simulink model "ControlComparison"  (R2018a)
settings: Solver=VariableStepAuto  StartTime=0  StopTime=4  FixedStep=1e-6
undefined symbols (not defined in the file): alternator, electrical_load, i_f_max, iceToAltRotRatio, n_ice_f, n_ice_i, normalizationFactor, rectifier, t_brake_f, t_brake_i, T_k, T_s
libraries: elec_lib x36, fl_lib x29, nesl_utility x26, neural x25, simulink x6, SimscapeCustomBlocks_lib x2
(part 2 of 3)

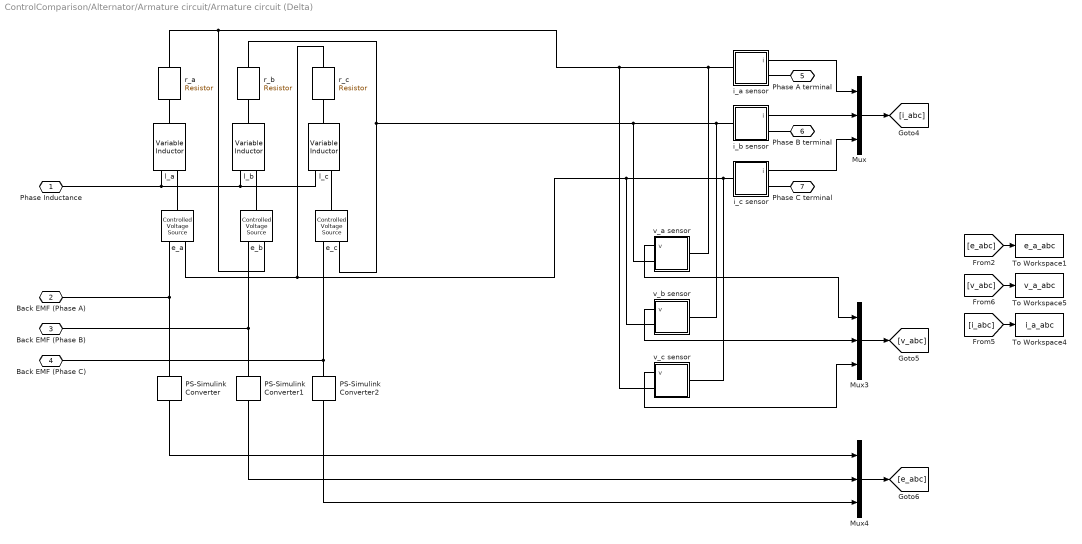
== system ControlComparison/Alternator/Armature circuit/Armature circuit (Delta) ==
  Mux : Mux  Inputs=3
  Mux3 : Mux  Inputs=3
  Mux4 : Mux  Inputs=3
  PS-Simulink Converter : nesl_utility/PS-Simulink Converter  PhysicalDomain=network_engine_domain  SubClassName=ps_output  LeftPortType=input  RightPortType=output  PseudoPeriodic=off  Frequencies=[]  Unit=1  AffineConversion=off
  PS-Simulink Converter1 : nesl_utility/PS-Simulink Converter  PhysicalDomain=network_engine_domain  SubClassName=ps_output  LeftPortType=input  RightPortType=output  PseudoPeriodic=off  Frequencies=[]  Unit=1  AffineConversion=off
  PS-Simulink Converter2 : nesl_utility/PS-Simulink Converter  PhysicalDomain=network_engine_domain  SubClassName=ps_output  LeftPortType=input  RightPortType=output  PseudoPeriodic=off  Frequencies=[]  Unit=1  AffineConversion=off
  To Workspace1 : ToWorkspace  VariableName=e_a_abc  SaveFormat=Timeseries  SampleTime=-1
  To Workspace4 : ToWorkspace  VariableName=i_a_abc  SaveFormat=Timeseries  SampleTime=-1
  To Workspace5 : ToWorkspace  VariableName=v_a_abc  SaveFormat=Timeseries  SampleTime=-1
  e_a : fl_lib/Electrical/Electrical Sources/Controlled Voltage Source
  e_b : fl_lib/Electrical/Electrical Sources/Controlled Voltage Source
  e_c : fl_lib/Electrical/Electrical Sources/Controlled Voltage Source
  i_a sensor : Subsystem
  i_b sensor : Subsystem
  i_c sensor : Subsystem
  l_a : elec_lib/Passive Devices/Variable Inductor  prm=1  Lmin=1e-6 H  g=1e-9 1/Ohm  i0=0 A  phi0=0 Wb
      settings: SourceProductName=Simscape Electronics  SourceProductBaseCode=SN
  l_b : elec_lib/Passive Devices/Variable Inductor  prm=1  Lmin=1e-6 H  g=1e-9 1/Ohm  i0=0 A  phi0=0 Wb
      settings: SourceProductName=Simscape Electronics  SourceProductBaseCode=SN
  l_c : elec_lib/Passive Devices/Variable Inductor  prm=1  Lmin=1e-6 H  g=1e-9 1/Ohm  i0=0 A  phi0=0 Wb
      settings: SourceProductName=Simscape Electronics  SourceProductBaseCode=SN
  r_a : elec_lib/Passive Devices/Resistor  R=alternator.stator.r.value Ohm  R_tol=5  enable_R_tol=0  tol_distribution=1  nSigma=4  enable_operating_limits=0  operating_limit_action=2  max_working_voltage=100 V  power_rating=1 W  enable_faults=0  fault_action=1  R_faulted=inf Ohm  enable_temporal_fault=0  t_fault=1 s  enable_behavioral_fault=0  max_permissible_current=1 A  t_fail_on_current=1 s  noise_mode=0  sample_time=1e-3 s  repeatability=1  auto_seed=4144164703  user_seed=0  Tdevice=25 degC  alpha=3.93e-3 1/K  Tmeas=25 degC  thermal_mass=100 J/K  power_derating_T1=70 degC  power_derating_T2=155 degC  operating_temperature_range_vec=[-50, 150] degC  temperature_specify=off  temperature_priority=High  temperature=298.15 K  temperature_nominal_specify=off  temperature_nominal_unit=K  temperature_nominal_value=1
  r_b : elec_lib/Passive Devices/Resistor  R=alternator.stator.r.value Ohm  R_tol=5  enable_R_tol=0  tol_distribution=1  nSigma=4  enable_operating_limits=0  operating_limit_action=2  max_working_voltage=100 V  power_rating=1 W  enable_faults=0  fault_action=1  R_faulted=inf Ohm  enable_temporal_fault=0  t_fault=1 s  enable_behavioral_fault=0  max_permissible_current=1 A  t_fail_on_current=1 s  noise_mode=0  sample_time=1e-3 s  repeatability=1  auto_seed=676943032  user_seed=0  Tdevice=25 degC  alpha=3.93e-3 1/K  Tmeas=25 degC  thermal_mass=100 J/K  power_derating_T1=70 degC  power_derating_T2=155 degC  operating_temperature_range_vec=[-50, 150] degC  temperature_specify=off  temperature_priority=High  temperature=298.15 K  temperature_nominal_specify=off  temperature_nominal_unit=K  temperature_nominal_value=1
  r_c : elec_lib/Passive Devices/Resistor  R=alternator.stator.r.value Ohm  R_tol=5  enable_R_tol=0  tol_distribution=1  nSigma=4  enable_operating_limits=0  operating_limit_action=2  max_working_voltage=100 V  power_rating=1 W  enable_faults=0  fault_action=1  R_faulted=inf Ohm  enable_temporal_fault=0  t_fault=1 s  enable_behavioral_fault=0  max_permissible_current=1 A  t_fail_on_current=1 s  noise_mode=0  sample_time=1e-3 s  repeatability=1  auto_seed=4168664255  user_seed=0  Tdevice=25 degC  alpha=3.93e-3 1/K  Tmeas=25 degC  thermal_mass=100 J/K  power_derating_T1=70 degC  power_derating_T2=155 degC  operating_temperature_range_vec=[-50, 150] degC  temperature_specify=off  temperature_priority=High  temperature=298.15 K  temperature_nominal_specify=off  temperature_nominal_unit=K  temperature_nominal_value=1
  v_a sensor : Subsystem
  v_b sensor : Subsystem
  v_c sensor : Subsystem
  Phase Inductance : PMIOPort  Side=Left
  Back EMF (Phase A) : PMIOPort  Port=2  Side=Left
  Back EMF (Phase B) : PMIOPort  Port=3  Side=Left
  Back EMF (Phase C) : PMIOPort  Port=4  Side=Left
  Phase A terminal : PMIOPort  Port=5  Side=Right
  Phase B terminal : PMIOPort  Port=6  Side=Right
  Phase C terminal : PMIOPort  Port=7  Side=Right
  wires:
  i_a sensor/1(i) -> Mux/1
  i_b sensor/1(i) -> Mux/2
  i_c sensor/1(i) -> Mux/3
  Mux/1 -> [i_abc]
  Mux3/1 -> [v_abc]
  v_b sensor/1(v) -> Mux3/2
  v_c sensor/1(v) -> Mux3/3
  v_a sensor/1(v) -> Mux3/1
  [i_abc] -> To Workspace4/1
  [v_abc] -> To Workspace5/1
  PS-Simulink Converter/1 -> Mux4/1
  PS-Simulink Converter1/1 -> Mux4/2
  PS-Simulink Converter2/1 -> Mux4/3
  Mux4/1 -> [e_abc]
  [e_abc] -> To Workspace1/1
  connections:
  i_a sensor/RConn1 -- Phase A terminal/RConn1
  Back EMF (Phase A)/RConn1 -- e_a/RConn1 -- PS-Simulink Converter/LConn1
  Back EMF (Phase B)/RConn1 -- e_b/RConn1 -- PS-Simulink Converter1/LConn1
  Back EMF (Phase C)/RConn1 -- e_c/RConn1 -- PS-Simulink Converter2/LConn1
  e_c/LConn1 -- l_c/LConn2
  e_b/LConn1 -- l_b/LConn2
  e_a/LConn1 -- l_a/LConn2
  r_c/LConn1 -- l_c/RConn1
  r_b/LConn1 -- l_b/RConn1
  r_a/LConn1 -- l_a/RConn1
  i_c sensor/RConn1 -- Phase C terminal/RConn1
  i_b sensor/RConn1 -- Phase B terminal/RConn1
  l_a/LConn1 -- Phase Inductance/RConn1 -- l_b/LConn1 -- l_c/LConn1
  e_b/RConn2 -- r_a/RConn1 -- v_a sensor/LConn1 -- i_a sensor/LConn1 -- v_c sensor/RConn1
  v_a sensor/RConn1 -- e_c/RConn2 -- r_b/RConn1 -- i_b sensor/LConn1 -- v_b sensor/LConn1
  r_c/RConn1 -- e_a/RConn2 -- v_c sensor/LConn1 -- i_c sensor/LConn1 -- v_b sensor/RConn1

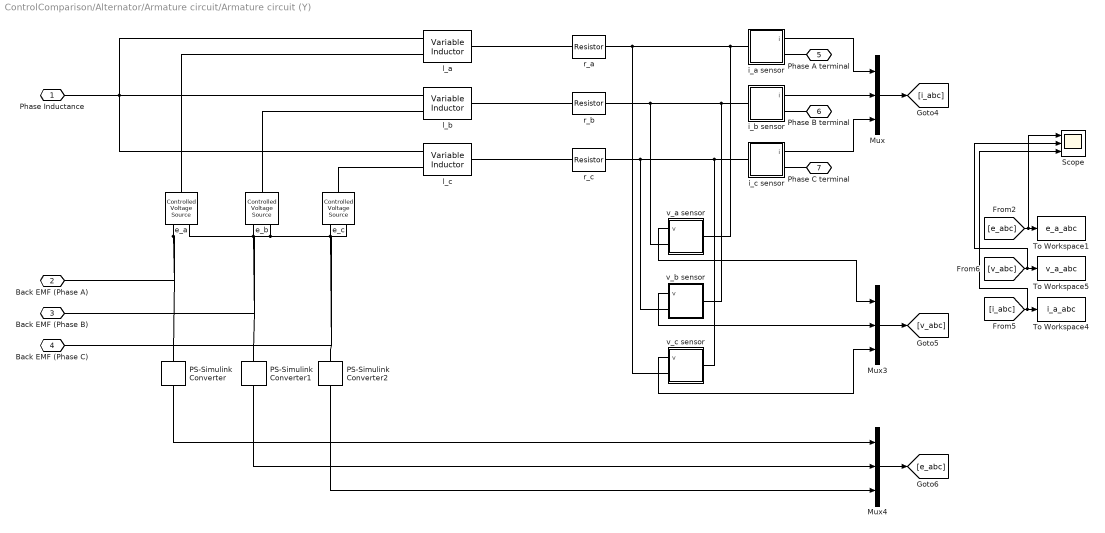
== system ControlComparison/Alternator/Armature circuit/Armature circuit (Y) ==
  Mux : Mux  Inputs=3
  Mux3 : Mux  Inputs=3
  Mux4 : Mux  Inputs=3
  PS-Simulink Converter : nesl_utility/PS-Simulink Converter  PhysicalDomain=network_engine_domain  SubClassName=ps_output  LeftPortType=input  RightPortType=output  PseudoPeriodic=off  Frequencies=[]  Unit=1  AffineConversion=off
  PS-Simulink Converter1 : nesl_utility/PS-Simulink Converter  PhysicalDomain=network_engine_domain  SubClassName=ps_output  LeftPortType=input  RightPortType=output  PseudoPeriodic=off  Frequencies=[]  Unit=1  AffineConversion=off
  PS-Simulink Converter2 : nesl_utility/PS-Simulink Converter  PhysicalDomain=network_engine_domain  SubClassName=ps_output  LeftPortType=input  RightPortType=output  PseudoPeriodic=off  Frequencies=[]  Unit=1  AffineConversion=off
  Scope : Scope  NumInputPorts=3
  To Workspace1 : ToWorkspace  VariableName=e_a_abc  SaveFormat=Timeseries  SampleTime=-1
  To Workspace4 : ToWorkspace  VariableName=i_a_abc  SaveFormat=Timeseries  SampleTime=-1
  To Workspace5 : ToWorkspace  VariableName=v_a_abc  SaveFormat=Timeseries  SampleTime=-1
  e_a : fl_lib/Electrical/Electrical Sources/Controlled Voltage Source
  e_b : fl_lib/Electrical/Electrical Sources/Controlled Voltage Source
  e_c : fl_lib/Electrical/Electrical Sources/Controlled Voltage Source
  i_a sensor : Subsystem
  i_b sensor : Subsystem
  i_c sensor : Subsystem
  l_a : elec_lib/Passive Devices/Variable Inductor  prm=1  Lmin=1e-6 H  g=1e-9 1/Ohm  i0=0 A  phi0=0 Wb
      settings: SourceProductName=Simscape Electronics  SourceProductBaseCode=SN
  l_b : elec_lib/Passive Devices/Variable Inductor  prm=1  Lmin=1e-6 H  g=1e-9 1/Ohm  i0=0 A  phi0=0 Wb
      settings: SourceProductName=Simscape Electronics  SourceProductBaseCode=SN
  l_c : elec_lib/Passive Devices/Variable Inductor  prm=1  Lmin=1e-6 H  g=1e-9 1/Ohm  i0=0 A  phi0=0 Wb
      settings: SourceProductName=Simscape Electronics  SourceProductBaseCode=SN
  r_a : elec_lib/Passive Devices/Resistor  R=alternator.stator.r.value/3 Ohm  R_tol=5  enable_R_tol=0  tol_distribution=1  nSigma=4  enable_operating_limits=0  operating_limit_action=2  max_working_voltage=100 V  power_rating=1 W  enable_faults=0  fault_action=1  R_faulted=inf Ohm  enable_temporal_fault=0  t_fault=1 s  enable_behavioral_fault=0  max_permissible_current=1 A  t_fail_on_current=1 s  noise_mode=0  sample_time=1e-3 s  repeatability=1  auto_seed=3922919431  user_seed=0  Tdevice=25 degC  alpha=3.93e-3 1/K  Tmeas=25 degC  thermal_mass=100 J/K  power_derating_T1=70 degC  power_derating_T2=155 degC  operating_temperature_range_vec=[-50, 150] degC  temperature_specify=off  temperature_priority=High  temperature=298.15 K  temperature_nominal_specify=off  temperature_nominal_unit=K  temperature_nominal_value=1
  r_b : elec_lib/Passive Devices/Resistor  R=alternator.stator.r.value/3 Ohm  R_tol=5  enable_R_tol=0  tol_distribution=1  nSigma=4  enable_operating_limits=0  operating_limit_action=2  max_working_voltage=100 V  power_rating=1 W  enable_faults=0  fault_action=1  R_faulted=inf Ohm  enable_temporal_fault=0  t_fault=1 s  enable_behavioral_fault=0  max_permissible_current=1 A  t_fail_on_current=1 s  noise_mode=0  sample_time=1e-3 s  repeatability=1  auto_seed=2715962282  user_seed=0  Tdevice=25 degC  alpha=3.93e-3 1/K  Tmeas=25 degC  thermal_mass=100 J/K  power_derating_T1=70 degC  power_derating_T2=155 degC  operating_temperature_range_vec=[-50, 150] degC  temperature_specify=off  temperature_priority=High  temperature=298.15 K  temperature_nominal_specify=off  temperature_nominal_unit=K  temperature_nominal_value=1
  r_c : elec_lib/Passive Devices/Resistor  R=alternator.stator.r.value/3 Ohm  R_tol=5  enable_R_tol=0  tol_distribution=1  nSigma=4  enable_operating_limits=0  operating_limit_action=2  max_working_voltage=100 V  power_rating=1 W  enable_faults=0  fault_action=1  R_faulted=inf Ohm  enable_temporal_fault=0  t_fault=1 s  enable_behavioral_fault=0  max_permissible_current=1 A  t_fail_on_current=1 s  noise_mode=0  sample_time=1e-3 s  repeatability=1  auto_seed=418932850  user_seed=0  Tdevice=25 degC  alpha=3.93e-3 1/K  Tmeas=25 degC  thermal_mass=100 J/K  power_derating_T1=70 degC  power_derating_T2=155 degC  operating_temperature_range_vec=[-50, 150] degC  temperature_specify=off  temperature_priority=High  temperature=298.15 K  temperature_nominal_specify=off  temperature_nominal_unit=K  temperature_nominal_value=1
  v_a sensor : Subsystem
  v_b sensor : Subsystem
  v_c sensor : Subsystem
  Phase Inductance : PMIOPort  Side=Left
  Back EMF (Phase A) : PMIOPort  Port=2  Side=Left
  Back EMF (Phase B) : PMIOPort  Port=3  Side=Left
  Back EMF (Phase C) : PMIOPort  Port=4  Side=Left
  Phase A terminal : PMIOPort  Port=5  Side=Right
  Phase B terminal : PMIOPort  Port=6  Side=Right
  Phase C terminal : PMIOPort  Port=7  Side=Right
  wires:
  i_a sensor/1(i) -> Mux/1
  i_b sensor/1(i) -> Mux/2
  i_c sensor/1(i) -> Mux/3
  Mux/1 -> [i_abc]
  Mux3/1 -> [v_abc]
  v_b sensor/1(v) -> Mux3/2
  v_c sensor/1(v) -> Mux3/3
  v_a sensor/1(v) -> Mux3/1
  [i_abc] -> Scope/3, To Workspace4/1
  [v_abc] -> Scope/2, To Workspace5/1
  PS-Simulink Converter/1 -> Mux4/1
  PS-Simulink Converter1/1 -> Mux4/2
  PS-Simulink Converter2/1 -> Mux4/3
  Mux4/1 -> [e_abc]
  [e_abc] -> Scope/1, To Workspace1/1
  connections:
  i_a sensor/RConn1 -- Phase A terminal/RConn1
  e_a/RConn2 -- e_c/RConn2 -- e_b/RConn2
  e_c/LConn1 -- l_c/LConn2
  e_b/LConn1 -- l_b/LConn2
  e_a/LConn1 -- l_a/LConn2
  r_c/LConn1 -- l_c/RConn1
  r_b/LConn1 -- l_b/RConn1
  r_a/LConn1 -- l_a/RConn1
  i_a sensor/LConn1 -- v_a sensor/LConn1 -- v_c sensor/RConn1 -- r_a/RConn1
  i_c sensor/RConn1 -- Phase C terminal/RConn1
  i_b sensor/RConn1 -- Phase B terminal/RConn1
  i_c sensor/LConn1 -- v_c sensor/LConn1 -- v_b sensor/RConn1 -- r_c/RConn1
  r_b/RConn1 -- v_a sensor/RConn1 -- v_b sensor/LConn1 -- i_b sensor/LConn1
  l_a/LConn1 -- Phase Inductance/RConn1 -- l_c/LConn1 -- l_b/LConn1
  e_a/RConn1 -- Back EMF (Phase A)/RConn1 -- PS-Simulink Converter/LConn1
  e_b/RConn1 -- Back EMF (Phase B)/RConn1 -- PS-Simulink Converter1/LConn1
  e_c/RConn1 -- Back EMF (Phase C)/RConn1 -- PS-Simulink Converter2/LConn1

== system ControlComparison/Alternator/Excitation circuit/Current sensor ==
  Current Sensor1 : fl_lib/Electrical/Electrical Sensors/Current Sensor
  PS-Simulink Converter1 : nesl_utility/PS-Simulink Converter  PhysicalDomain=network_engine_domain  SubClassName=ps_output  LeftPortType=input  RightPortType=output  PseudoPeriodic=off  Frequencies=[]  Unit=1  AffineConversion=off
  Sample delay : TransferFcn  Denominator=[T_s 1]
  + : PMIOPort  Side=Left
  - : PMIOPort  Port=2  Side=Right
  i (PS) : PMIOPort  Port=3  Side=Right
  i (Sim) : Outport
  wires:
  Sample delay/1 -> i (Sim)/1
  PS-Simulink Converter1/1 -> Sample delay/1
  connections:
  Current Sensor1/RConn2 -- -/RConn1
  Current Sensor1/LConn1 -- +/RConn1
  PS-Simulink Converter1/LConn1 -- i (PS)/RConn1 -- Current Sensor1/RConn1

== system ControlComparison/Alternator/Excitation circuit/Driver ==
  Controlled PWM Voltage : elec_lib/Actuators & Drivers/Drivers/Controlled PWM Voltage  F=alternator.rotor.control.pwm.f_s Hz  TD=0 s  pulse_width_offset=0 s  pulse_min=0 s  Vmin=0 V  Vmax=5 V  Vm=5 V  pwm_or_av=1  event_type=2  sample_time=T_s s  u_min=0  u_max=1
      settings: SourceProductName=Simscape Electronics  SourceProductBaseCode=SN  LogSimulationData=on
  Electrical Reference : fl_lib/Electrical/Electrical Elements/Electrical Reference
  Gate Driver : elec_lib/Actuators & Drivers/Drivers/Gate Driver  vHigh=rectifier.s.v_gs_on*1.5 V  vLow=0 V  parameterization=1  rHigh=100 Ohm  rLow=10 Ohm  tRise=20 ns  tFall=20 ns  cLoad=10 nF  enable_faults=0  t_fault=1 s  fault_type=1  uHighValue=0.7  uLowValue=0.3  tHigh=50 ns  tLow=100 ns  ZonTime_specify=off  ZonTime_priority=None  ZonTime=0 s  ZoffTime_specify=off  ZoffTime_priority=None  ZoffTime=0 s  uHigh=2.0 V  uLow=0.8 V
      settings: SourceProductName=Simscape Electronics  SourceProductBaseCode=SN  LogSimulationData=on
  d : PMIOPort  Side=Left
  v_g : PMIOPort  Port=2  Side=Right
  v_s : PMIOPort  Port=3  Side=Right
  connections:
  Gate Driver/LConn2 -- Electrical Reference/LConn1 -- Controlled PWM Voltage/RConn2
  Controlled PWM Voltage/RConn1 -- Gate Driver/LConn1
  v_g/RConn1 -- Gate Driver/RConn1
  v_s/RConn1 -- Gate Driver/RConn2
  d/RConn1 -- Controlled PWM Voltage/LConn1

== system ControlComparison/Control scheme/Conventional Control Scheme/Excitation current controller ==
  e : Inport
  on : Inport  Port=2
  Constant : Constant
  Fcn : Fcn  Expr=u > 0
  Switch : Switch  Criteria=u2 > Threshold  Threshold=0.5
  u : Outport
  wires:
  Switch/1 -> u/1
  on/1 -> Switch/2
  Constant/1 -> Switch/3
  Fcn/1 -> Switch/1
  e/1 -> Fcn/1

== system ControlComparison/Control scheme/Full Excitation Current Control Scheme/Excitation current controller ==
  e : Inport
  on : Inport  Port=2
  Constant : Constant
  Fcn : Fcn  Expr=u > 0
  Switch : Switch  Criteria=u2 > Threshold  Threshold=0.5
  u : Outport
  wires:
  Switch/1 -> u/1
  on/1 -> Switch/2
  Constant/1 -> Switch/3
  Fcn/1 -> Switch/1
  e/1 -> Fcn/1

== system ControlComparison/Control scheme/Neural MPPT Control Scheme/Excitation current controller ==
  e : Inport
  on : Inport  Port=2
  Constant : Constant
  Fcn : Fcn  Expr=u > 0
  Switch : Switch  Criteria=u2 > Threshold  Threshold=0.5
  u : Outport
  wires:
  Switch/1 -> u/1
  on/1 -> Switch/2
  Constant/1 -> Switch/3
  Fcn/1 -> Switch/1
  e/1 -> Fcn/1

== system ControlComparison/Control scheme/Neural MPPT Control Scheme/Mapped Duty Cycle Neural Controller ==
  Input : Inport  PortDimensions=3
      mask Display: e = 0.06;c1 = [120 230 180]/255;c2 = ([120 230 180]+0)/(256+128);c3 = ([120 230 180]+128)/(256+128);patch([0 1 1 0],[0 0 1 1],c1);patch([0 1 1 1-e 1-e 0+e],[0 0 1 1-e 0+e 0+e],c2);patch([0 0 1 1-e 0+e 0+e],[0 1 1 1-e 1-e 0+e],c3);plot([0 1 1 0 0],[0 0 1 1 0]);
  Layer 1 : Subsystem
      mask Display: e = 0.06;c1 = [120 150 230]/255;c2 = ([120 150 230]+0)/383;c3 = ([120 150 230]+128)/383;patch([0 1 1 0],[0 0 1 1],c1);patch([0 1 1 1-e 1-e 0+e],[0 0 1 1-e 0+e 0+e],c2);patch([0 0 1 1-e 0+e 0+e],[0 1 1 1-e 1-e 0+e],c3);plot([0 1 1 0 0],[0 0 1 1 0]);
  Layer 2 : Subsystem
      mask Display: e = 0.06;c1 = [120 150 230]/255;c2 = ([120 150 230]+0)/383;c3 = ([120 150 230]+128)/383;patch([0 1 1 0],[0 0 1 1],c1);patch([0 1 1 1-e 1-e 0+e],[0 0 1 1-e 0+e 0+e],c2);patch([0 0 1 1-e 0+e 0+e],[0 1 1 1-e 1-e 0+e],c3);plot([0 1 1 0 0],[0 0 1 1 0]);
  Process Input 1 : Subsystem
      mask Display: e = 0.06;c1 = [120 150 230]/255;c2 = ([120 150 230]+0)/383;c3 = ([120 150 230]+128)/383;patch([0 1 1 0],[0 0 1 1],c1);patch([0 1 1 1-e 1-e 0+e],[0 0 1 1-e 0+e 0+e],c2);patch([0 0 1 1-e 0+e 0+e],[0 1 1 1-e 1-e 0+e],c3);plot([0 1 1 0 0],[0 0 1 1 0]);
  Process Output 1 : Subsystem
      mask Display: e = 0.06;c1 = [120 150 230]/255;c2 = ([120 150 230]+0)/383;c3 = ([120 150 230]+128)/383;patch([0 1 1 0],[0 0 1 1],c1);patch([0 1 1 1-e 1-e 0+e],[0 0 1 1-e 0+e 0+e],c2);patch([0 0 1 1-e 0+e 0+e],[0 1 1 1-e 1-e 0+e],c3);plot([0 1 1 0 0],[0 0 1 1 0]);
  Output : Outport  InitialOutput=0
      mask Display: e = 0.06;c1 = [120 230 180]/255;c2 = ([120 230 180]+0)/(256+128);c3 = ([120 230 180]+128)/(256+128);patch([0 1 1 0],[0 0 1 1],c1);patch([0 1 1 1-e 1-e 0+e],[0 0 1 1-e 0+e 0+e],c2);patch([0 0 1 1-e 0+e 0+e],[0 1 1 1-e 1-e 0+e],c3);plot([0 1 1 0 0],[0 0 1 1 0]);
  wires:
  Layer 2/1("a{2}") -> Process Output 1/1(a)
  [feedback1] -> Layer 2/1("a{1} ")
  Layer 1/1("a{1}") -> [feedback1]
  Process Input 1/1(p) -> Layer 1/1("p{1}")
  Process Output 1/1(y) -> Output/1
  Input/1 -> Process Input 1/1(x)

== system ControlComparison/i_l sensor/Current Sensor/Ideal current sensor ==
  Current Sensor : fl_lib/Electrical/Electrical Sensors/Current Sensor
  PS-Simulink Converter : nesl_utility/PS-Simulink Converter  PhysicalDomain=network_engine_domain  SubClassName=ps_output  LeftPortType=input  RightPortType=output  PseudoPeriodic=off  Frequencies=[]  Unit=1  AffineConversion=off
  + : PMIOPort  Side=Left
  - : PMIOPort  Port=2  Side=Right
  i : Outport
  wires:
  PS-Simulink Converter/1 -> i/1
  connections:
  Current Sensor/RConn2 -- -/RConn1
  Current Sensor/LConn1 -- +/RConn1
  PS-Simulink Converter/LConn1 -- Current Sensor/RConn1

== system ControlComparison/i_l sensor/Current Sensor/Noise addition ==
  u : Inport
  Band-Limited White Noise : simulink/Sources/Band-Limited White Noise  Cov=[0.1]  Ts=T_s  seed=[seed]
  Gain : Gain  Gain=1/100
  Gain3 : Gain  Gain=noise
  Product2 : Product
  Sum1 : Sum  Inputs=|++
  Zero-Order Hold : ZeroOrderHold  SampleTime=T_s
  u + n : Outport
  wires:
  Gain3/1 -> Product2/1
  Product2/1 -> Sum1/1
  Gain/1 -> Product2/2
  u/1 -> Sum1/2, Gain3/1
  Band-Limited White Noise/1 -> Gain/1
  Sum1/1 -> Zero-Order Hold/1
  Zero-Order Hold/1 -> u + n/1

== system ControlComparison/v_b sensor/Voltage Sensor/Ideal voltage sensor ==
  PS-Simulink Converter : nesl_utility/PS-Simulink Converter  PhysicalDomain=network_engine_domain  SubClassName=ps_output  LeftPortType=input  RightPortType=output  PseudoPeriodic=off  Frequencies=[]  Unit=1  AffineConversion=off
  Voltage Sensor : fl_lib/Electrical/Electrical Sensors/Voltage Sensor
  + : PMIOPort  Side=Left
  - : PMIOPort  Port=2  Side=Right
  v : Outport
  wires:
  PS-Simulink Converter/1 -> v/1
  connections:
  Voltage Sensor/LConn1 -- +/RConn1
  -/RConn1 -- Voltage Sensor/RConn2
  Voltage Sensor/RConn1 -- PS-Simulink Converter/LConn1

== system ControlComparison/v_b sensor/Voltage Sensor/Noise addition ==
  u : Inport
  Band-Limited White Noise : simulink/Sources/Band-Limited White Noise  Cov=[0.1]  Ts=T_s  seed=[seed]
  Gain : Gain  Gain=1/100
  Gain3 : Gain  Gain=noise
  Product2 : Product
  Sum1 : Sum  Inputs=|++
  Zero-Order Hold : ZeroOrderHold  SampleTime=T_s
  u + n : Outport
  wires:
  Gain3/1 -> Product2/1
  Product2/1 -> Sum1/1
  Gain/1 -> Product2/2
  u/1 -> Sum1/2, Gain3/1
  Band-Limited White Noise/1 -> Gain/1
  Sum1/1 -> Zero-Order Hold/1
  Zero-Order Hold/1 -> u + n/1

== system ControlComparison/v_l sensor/Voltage Sensor/Ideal voltage sensor ==
  PS-Simulink Converter : nesl_utility/PS-Simulink Converter  PhysicalDomain=network_engine_domain  SubClassName=ps_output  LeftPortType=input  RightPortType=output  PseudoPeriodic=off  Frequencies=[]  Unit=1  AffineConversion=off
  Voltage Sensor : fl_lib/Electrical/Electrical Sensors/Voltage Sensor
  + : PMIOPort  Side=Left
  - : PMIOPort  Port=2  Side=Right
  v : Outport
  wires:
  PS-Simulink Converter/1 -> v/1
  connections:
  Voltage Sensor/LConn1 -- +/RConn1
  -/RConn1 -- Voltage Sensor/RConn2
  Voltage Sensor/RConn1 -- PS-Simulink Converter/LConn1

== system ControlComparison/v_l sensor/Voltage Sensor/Noise addition ==
  u : Inport
  Band-Limited White Noise : simulink/Sources/Band-Limited White Noise  Cov=[0.1]  Ts=T_s  seed=[seed]
  Gain : Gain  Gain=1/100
  Gain3 : Gain  Gain=noise
  Product2 : Product
  Sum1 : Sum  Inputs=|++
  Zero-Order Hold : ZeroOrderHold  SampleTime=T_s
  u + n : Outport
  wires:
  Gain3/1 -> Product2/1
  Product2/1 -> Sum1/1
  Gain/1 -> Product2/2
  u/1 -> Sum1/2, Gain3/1
  Band-Limited White Noise/1 -> Gain/1
  Sum1/1 -> Zero-Order Hold/1
  Zero-Order Hold/1 -> u + n/1

== system ControlComparison/Alternator/Armature circuit/Armature circuit (Delta)/i_a sensor ==
  Current Sensor : fl_lib/Electrical/Electrical Sensors/Current Sensor
  PS-Simulink Converter : nesl_utility/PS-Simulink Converter  PhysicalDomain=network_engine_domain  SubClassName=ps_output  LeftPortType=input  RightPortType=output  PseudoPeriodic=off  Frequencies=[]  Unit=1  AffineConversion=off
  + : PMIOPort  Side=Left
  - : PMIOPort  Port=2  Side=Right
  i : Outport
  wires:
  PS-Simulink Converter/1 -> i/1
  connections:
  Current Sensor/RConn2 -- -/RConn1
  Current Sensor/LConn1 -- +/RConn1
  PS-Simulink Converter/LConn1 -- Current Sensor/RConn1

== system ControlComparison/Alternator/Armature circuit/Armature circuit (Delta)/i_b sensor ==
  Current Sensor : fl_lib/Electrical/Electrical Sensors/Current Sensor
  PS-Simulink Converter : nesl_utility/PS-Simulink Converter  PhysicalDomain=network_engine_domain  SubClassName=ps_output  LeftPortType=input  RightPortType=output  PseudoPeriodic=off  Frequencies=[]  Unit=1  AffineConversion=off
  + : PMIOPort  Side=Left
  - : PMIOPort  Port=2  Side=Right
  i : Outport
  wires:
  PS-Simulink Converter/1 -> i/1
  connections:
  Current Sensor/RConn2 -- -/RConn1
  Current Sensor/LConn1 -- +/RConn1
  PS-Simulink Converter/LConn1 -- Current Sensor/RConn1

== system ControlComparison/Alternator/Armature circuit/Armature circuit (Delta)/i_c sensor ==
  Current Sensor : fl_lib/Electrical/Electrical Sensors/Current Sensor
  PS-Simulink Converter : nesl_utility/PS-Simulink Converter  PhysicalDomain=network_engine_domain  SubClassName=ps_output  LeftPortType=input  RightPortType=output  PseudoPeriodic=off  Frequencies=[]  Unit=1  AffineConversion=off
  + : PMIOPort  Side=Left
  - : PMIOPort  Port=2  Side=Right
  i : Outport
  wires:
  PS-Simulink Converter/1 -> i/1
  connections:
  Current Sensor/RConn2 -- -/RConn1
  Current Sensor/LConn1 -- +/RConn1
  PS-Simulink Converter/LConn1 -- Current Sensor/RConn1

== system ControlComparison/Alternator/Armature circuit/Armature circuit (Delta)/v_a sensor ==
  PS-Simulink Converter : nesl_utility/PS-Simulink Converter  PhysicalDomain=network_engine_domain  SubClassName=ps_output  LeftPortType=input  RightPortType=output  PseudoPeriodic=off  Frequencies=[]  Unit=1  AffineConversion=off
  Voltage Sensor : fl_lib/Electrical/Electrical Sensors/Voltage Sensor
  + : PMIOPort  Side=Left
  - : PMIOPort  Port=2  Side=Right
  v : Outport
  wires:
  PS-Simulink Converter/1 -> v/1
  connections:
  Voltage Sensor/LConn1 -- +/RConn1
  -/RConn1 -- Voltage Sensor/RConn2
  Voltage Sensor/RConn1 -- PS-Simulink Converter/LConn1

== system ControlComparison/Alternator/Armature circuit/Armature circuit (Delta)/v_b sensor ==
  PS-Simulink Converter : nesl_utility/PS-Simulink Converter  PhysicalDomain=network_engine_domain  SubClassName=ps_output  LeftPortType=input  RightPortType=output  PseudoPeriodic=off  Frequencies=[]  Unit=1  AffineConversion=off
  Voltage Sensor : fl_lib/Electrical/Electrical Sensors/Voltage Sensor
  + : PMIOPort  Side=Left
  - : PMIOPort  Port=2  Side=Right
  v : Outport
  wires:
  PS-Simulink Converter/1 -> v/1
  connections:
  Voltage Sensor/LConn1 -- +/RConn1
  -/RConn1 -- Voltage Sensor/RConn2
  Voltage Sensor/RConn1 -- PS-Simulink Converter/LConn1

== system ControlComparison/Alternator/Armature circuit/Armature circuit (Delta)/v_c sensor ==
  PS-Simulink Converter : nesl_utility/PS-Simulink Converter  PhysicalDomain=network_engine_domain  SubClassName=ps_output  LeftPortType=input  RightPortType=output  PseudoPeriodic=off  Frequencies=[]  Unit=1  AffineConversion=off
  Voltage Sensor : fl_lib/Electrical/Electrical Sensors/Voltage Sensor
  + : PMIOPort  Side=Left
  - : PMIOPort  Port=2  Side=Right
  v : Outport
  wires:
  PS-Simulink Converter/1 -> v/1
  connections:
  Voltage Sensor/LConn1 -- +/RConn1
  -/RConn1 -- Voltage Sensor/RConn2
  Voltage Sensor/RConn1 -- PS-Simulink Converter/LConn1

== system ControlComparison/Alternator/Armature circuit/Armature circuit (Y)/i_a sensor ==
  Current Sensor : fl_lib/Electrical/Electrical Sensors/Current Sensor
  PS-Simulink Converter : nesl_utility/PS-Simulink Converter  PhysicalDomain=network_engine_domain  SubClassName=ps_output  LeftPortType=input  RightPortType=output  PseudoPeriodic=off  Frequencies=[]  Unit=1  AffineConversion=off
  + : PMIOPort  Side=Left
  - : PMIOPort  Port=2  Side=Right
  i : Outport
  wires:
  PS-Simulink Converter/1 -> i/1
  connections:
  Current Sensor/RConn2 -- -/RConn1
  Current Sensor/LConn1 -- +/RConn1
  PS-Simulink Converter/LConn1 -- Current Sensor/RConn1

== system ControlComparison/Alternator/Armature circuit/Armature circuit (Y)/i_b sensor ==
  Current Sensor : fl_lib/Electrical/Electrical Sensors/Current Sensor
  PS-Simulink Converter : nesl_utility/PS-Simulink Converter  PhysicalDomain=network_engine_domain  SubClassName=ps_output  LeftPortType=input  RightPortType=output  PseudoPeriodic=off  Frequencies=[]  Unit=1  AffineConversion=off
  + : PMIOPort  Side=Left
  - : PMIOPort  Port=2  Side=Right
  i : Outport
  wires:
  PS-Simulink Converter/1 -> i/1
  connections:
  Current Sensor/RConn2 -- -/RConn1
  Current Sensor/LConn1 -- +/RConn1
  PS-Simulink Converter/LConn1 -- Current Sensor/RConn1

== system ControlComparison/Alternator/Armature circuit/Armature circuit (Y)/i_c sensor ==
  Current Sensor : fl_lib/Electrical/Electrical Sensors/Current Sensor
  PS-Simulink Converter : nesl_utility/PS-Simulink Converter  PhysicalDomain=network_engine_domain  SubClassName=ps_output  LeftPortType=input  RightPortType=output  PseudoPeriodic=off  Frequencies=[]  Unit=1  AffineConversion=off
  + : PMIOPort  Side=Left
  - : PMIOPort  Port=2  Side=Right
  i : Outport
  wires:
  PS-Simulink Converter/1 -> i/1
  connections:
  Current Sensor/RConn2 -- -/RConn1
  Current Sensor/LConn1 -- +/RConn1
  PS-Simulink Converter/LConn1 -- Current Sensor/RConn1

== system ControlComparison/Alternator/Armature circuit/Armature circuit (Y)/v_a sensor ==
  PS-Simulink Converter : nesl_utility/PS-Simulink Converter  PhysicalDomain=network_engine_domain  SubClassName=ps_output  LeftPortType=input  RightPortType=output  PseudoPeriodic=off  Frequencies=[]  Unit=1  AffineConversion=off
  Voltage Sensor : fl_lib/Electrical/Electrical Sensors/Voltage Sensor
  + : PMIOPort  Side=Left
  - : PMIOPort  Port=2  Side=Right
  v : Outport
  wires:
  PS-Simulink Converter/1 -> v/1
  connections:
  Voltage Sensor/LConn1 -- +/RConn1
  -/RConn1 -- Voltage Sensor/RConn2
  Voltage Sensor/RConn1 -- PS-Simulink Converter/LConn1

== system ControlComparison/Alternator/Armature circuit/Armature circuit (Y)/v_b sensor ==
  PS-Simulink Converter : nesl_utility/PS-Simulink Converter  PhysicalDomain=network_engine_domain  SubClassName=ps_output  LeftPortType=input  RightPortType=output  PseudoPeriodic=off  Frequencies=[]  Unit=1  AffineConversion=off
  Voltage Sensor : fl_lib/Electrical/Electrical Sensors/Voltage Sensor
  + : PMIOPort  Side=Left
  - : PMIOPort  Port=2  Side=Right
  v : Outport
  wires:
  PS-Simulink Converter/1 -> v/1
  connections:
  Voltage Sensor/LConn1 -- +/RConn1
  -/RConn1 -- Voltage Sensor/RConn2
  Voltage Sensor/RConn1 -- PS-Simulink Converter/LConn1

== system ControlComparison/Alternator/Armature circuit/Armature circuit (Y)/v_c sensor ==
  PS-Simulink Converter : nesl_utility/PS-Simulink Converter  PhysicalDomain=network_engine_domain  SubClassName=ps_output  LeftPortType=input  RightPortType=output  PseudoPeriodic=off  Frequencies=[]  Unit=1  AffineConversion=off
  Voltage Sensor : fl_lib/Electrical/Electrical Sensors/Voltage Sensor
  + : PMIOPort  Side=Left
  - : PMIOPort  Port=2  Side=Right
  v : Outport
  wires:
  PS-Simulink Converter/1 -> v/1
  connections:
  Voltage Sensor/LConn1 -- +/RConn1
  -/RConn1 -- Voltage Sensor/RConn2
  Voltage Sensor/RConn1 -- PS-Simulink Converter/LConn1

== system ControlComparison/Control scheme/Neural MPPT Control Scheme/Mapped Duty Cycle Neural Controller/Layer 1 ==
  "p{1}" : Inport  PortDimensions=3
      mask Display: e = 0.06;c1 = [120 230 180]/255;c2 = ([120 230 180]+0)/(256+128);c3 = ([120 230 180]+128)/(256+128);patch([0 1 1 0],[0 0 1 1],c1);patch([0 1 1 1-e 1-e 0+e],[0 0 1 1-e 0+e 0+e],c2);patch([0 0 1 1-e 0+e 0+e],[0 1 1 1-e 1-e 0+e],c3);plot([0 1 1 0 0],[0 0 1 1 0]);
  Delays 1 : Subsystem
      mask Display: e = 0.06;c1 = [120 150 230]/255;c2 = ([120 150 230]+0)/383;c3 = ([120 150 230]+128)/383;patch([0 1 1 0],[0 0 1 1],c1);patch([0 1 1 1-e 1-e 0+e],[0 0 1 1-e 0+e 0+e],c2);patch([0 0 1 1-e 0+e 0+e],[0 1 1 1-e 1-e 0+e],c3);plot([0 1 1 0 0],[0 0 1 1 0]);disp('0');
  "IW{1,1}" : Subsystem
      mask Display: e = 0.06;c1 = [120 150 230]/255;c2 = ([120 150 230]+0)/383;c3 = ([120 150 230]+128)/383;patch([0 1 1 0],[0 0 1 1],c1);patch([0 1 1 1-e 1-e 0+e],[0 0 1 1-e 0+e 0+e],c2);patch([0 0 1 1-e 0+e 0+e],[0 1 1 1-e 1-e 0+e],c3);plot([0 1 1 0 0],[0 0 1 1 0]);disp('W');
  "b{1}" : Constant  Value=[-7.74347657151980595102713778032921254634857177734375;-0.7897127108803854156349188997410237789154052734375;-20.200891871771347041430999524891376495361328125;-2.719102245714753340877223308780230581760406494140625;-17.07885408293710582938729203306138515472412109375;-10.049782933722664068909580237232148647308349609375;10.210016176689123312826268374919891357421875;4.3787125129864676864599459804594516754150390625;-20.6767216009456404890443081967532634735107421875;-6.69520556633330254925340341287665069103240966796875;21.80305946231902680665371008217334747314453125;5.45826406753966519858067840686999261379241943359375;2.921135354700396646876470185816287994384765625;-1.6904984852896338676231380304670892655849456787109375;-16.14727074386085092783105210401117801666259765625;-5.89151276233954401817527468665502965450286865234375;-2.474568326195348166862686412059701979160308837890625;-2.766773748500481300283126984140835702419281005859375;-7.02665483439283367061989338253624737262725830078125;18.97206346240232477384779485873878002166748046875]
      mask Display: e = 0.06;c1 = [120 150 230]/255;c2 = ([120 150 230]+0)/383;c3 = ([120 150 230]+128)/383;patch([0 1 1 0],[0 0 1 1],c1);patch([0 1 1 1-e 1-e 0+e],[0 0 1 1-e 0+e 0+e],c2);patch([0 0 1 1-e 0+e 0+e],[0 1 1 1-e 1-e 0+e],c3);plot([0 1 1 0 0],[0 0 1 1 0]);disp('b');
  netsum : Sum  Inputs=2  SaturateOnIntegerOverflow=on  InputSameDT=on  OutDataTypeStr=Inherit: Same as first input
      mask Display: e = 0.06;c1 = [120 150 230]/255;c2 = ([120 150 230]+0)/383;c3 = ([120 150 230]+128)/383;patch([0 1 1 0],[0 0 1 1],c1);patch([0 1 1 1-e 1-e 0+e],[0 0 1 1-e 0+e 0+e],c2);patch([0 0 1 1-e 0+e 0+e],[0 1 1 1-e 1-e 0+e],c3);plot([0 1 1 0 0],[0 0 1 1 0]);disp('+');
  tansig : neural/Transfer Functions/tansig
      settings: SourceProductName=Deep Learning Toolbox
  "a{1}" : Outport  InitialOutput=[0;0;0;0;0;0;0;0;0;0;0;0;0;0;0;0;0;0;0;0]
      mask Display: e = 0.06;c1 = [120 230 180]/255;c2 = ([120 230 180]+0)/(256+128);c3 = ([120 230 180]+128)/(256+128);patch([0 1 1 0],[0 0 1 1],c1);patch([0 1 1 1-e 1-e 0+e],[0 0 1 1-e 0+e 0+e],c2);patch([0 0 1 1-e 0+e 0+e],[0 1 1 1-e 1-e 0+e],c3);plot([0 1 1 0 0],[0 0 1 1 0]);
  wires:
  tansig/1 -> "a{1}"/1
  netsum/1 -> tansig/1
  "b{1}"/1 -> netsum/2
  "IW{1,1}"/1("iz{1,1}") -> netsum/1
  Delays 1/1("pd{1,1}") -> "IW{1,1}"/1("pd{1,1}")
  "p{1}"/1 -> Delays 1/1("p{1}")

== system ControlComparison/Control scheme/Neural MPPT Control Scheme/Mapped Duty Cycle Neural Controller/Layer 2 ==
  "a{1} " : Inport  PortDimensions=20
      mask Display: e = 0.06;c1 = [120 230 180]/255;c2 = ([120 230 180]+0)/(256+128);c3 = ([120 230 180]+128)/(256+128);patch([0 1 1 0],[0 0 1 1],c1);patch([0 1 1 1-e 1-e 0+e],[0 0 1 1-e 0+e 0+e],c2);patch([0 0 1 1-e 0+e 0+e],[0 1 1 1-e 1-e 0+e],c3);plot([0 1 1 0 0],[0 0 1 1 0]);
  Delays 1 : Subsystem
      mask Display: e = 0.06;c1 = [120 150 230]/255;c2 = ([120 150 230]+0)/383;c3 = ([120 150 230]+128)/383;patch([0 1 1 0],[0 0 1 1],c1);patch([0 1 1 1-e 1-e 0+e],[0 0 1 1-e 0+e 0+e],c2);patch([0 0 1 1-e 0+e 0+e],[0 1 1 1-e 1-e 0+e],c3);plot([0 1 1 0 0],[0 0 1 1 0]);disp('0');
  "LW{2,1}" : Subsystem
      mask Display: e = 0.06;c1 = [120 150 230]/255;c2 = ([120 150 230]+0)/383;c3 = ([120 150 230]+128)/383;patch([0 1 1 0],[0 0 1 1],c1);patch([0 1 1 1-e 1-e 0+e],[0 0 1 1-e 0+e 0+e],c2);patch([0 0 1 1-e 0+e 0+e],[0 1 1 1-e 1-e 0+e],c3);plot([0 1 1 0 0],[0 0 1 1 0]);disp('W');
  "b{2}" : Constant  Value=1.72889346041095581796298574772663414478302001953125
      mask Display: e = 0.06;c1 = [120 150 230]/255;c2 = ([120 150 230]+0)/383;c3 = ([120 150 230]+128)/383;patch([0 1 1 0],[0 0 1 1],c1);patch([0 1 1 1-e 1-e 0+e],[0 0 1 1-e 0+e 0+e],c2);patch([0 0 1 1-e 0+e 0+e],[0 1 1 1-e 1-e 0+e],c3);plot([0 1 1 0 0],[0 0 1 1 0]);disp('b');
  netsum : Sum  Inputs=2  SaturateOnIntegerOverflow=on  InputSameDT=on  OutDataTypeStr=Inherit: Same as first input
      mask Display: e = 0.06;c1 = [120 150 230]/255;c2 = ([120 150 230]+0)/383;c3 = ([120 150 230]+128)/383;patch([0 1 1 0],[0 0 1 1],c1);patch([0 1 1 1-e 1-e 0+e],[0 0 1 1-e 0+e 0+e],c2);patch([0 0 1 1-e 0+e 0+e],[0 1 1 1-e 1-e 0+e],c3);plot([0 1 1 0 0],[0 0 1 1 0]);disp('+');
  purelin : neural/Transfer Functions/purelin
      settings: SourceProductName=Deep Learning Toolbox
  "a{2}" : Outport  InitialOutput=0
      mask Display: e = 0.06;c1 = [120 230 180]/255;c2 = ([120 230 180]+0)/(256+128);c3 = ([120 230 180]+128)/(256+128);patch([0 1 1 0],[0 0 1 1],c1);patch([0 1 1 1-e 1-e 0+e],[0 0 1 1-e 0+e 0+e],c2);patch([0 0 1 1-e 0+e 0+e],[0 1 1 1-e 1-e 0+e],c3);plot([0 1 1 0 0],[0 0 1 1 0]);
  wires:
  purelin/1 -> "a{2}"/1
  netsum/1 -> purelin/1
  "b{2}"/1 -> netsum/2
  "LW{2,1}"/1("lz{2,1}") -> netsum/1
  Delays 1/1("pd{2,1}") -> "LW{2,1}"/1("ad{2,1}")
  "a{1} "/1 -> Delays 1/1("p{2}")

== system ControlComparison/Control scheme/Neural MPPT Control Scheme/Mapped Duty Cycle Neural Controller/Process Input 1 ==
  x : Inport  PortDimensions=3
      mask Display: e = 0.06;c1 = [120 230 180]/255;c2 = ([120 230 180]+0)/(256+128);c3 = ([120 230 180]+128)/(256+128);patch([0 1 1 0],[0 0 1 1],c1);patch([0 1 1 1-e 1-e 0+e],[0 0 1 1-e 0+e 0+e],c2);patch([0 0 1 1-e 0+e 0+e],[0 1 1 1-e 1-e 0+e],c3);plot([0 1 1 0 0],[0 0 1 1 0]);
  mapminmax : neural/Processing Functions/mapminmax  xmin=[0.0025000000000000000520417042793;0.25;0.00500000000000000010408340855861]  xmax=[1;1;1]  ymin=-1  ymax=1
      settings: SourceProductName=Deep Learning Toolbox
  p : Outport  PortDimensions=3
      mask Display: e = 0.06;c1 = [120 230 180]/255;c2 = ([120 230 180]+0)/(256+128);c3 = ([120 230 180]+128)/(256+128);patch([0 1 1 0],[0 0 1 1],c1);patch([0 1 1 1-e 1-e 0+e],[0 0 1 1-e 0+e 0+e],c2);patch([0 0 1 1-e 0+e 0+e],[0 1 1 1-e 1-e 0+e],c3);plot([0 1 1 0 0],[0 0 1 1 0]);
  wires:
  mapminmax/1 -> p/1
  x/1 -> mapminmax/1

== system ControlComparison/Control scheme/Neural MPPT Control Scheme/Mapped Duty Cycle Neural Controller/Process Output 1 ==
  a : Inport  PortDimensions=1
      mask Display: e = 0.06;c1 = [120 230 180]/255;c2 = ([120 230 180]+0)/(256+128);c3 = ([120 230 180]+128)/(256+128);patch([0 1 1 0],[0 0 1 1],c1);patch([0 1 1 1-e 1-e 0+e],[0 0 1 1-e 0+e 0+e],c2);patch([0 0 1 1-e 0+e 0+e],[0 1 1 1-e 1-e 0+e],c3);plot([0 1 1 0 0],[0 0 1 1 0]);
  mapminmax_reverse : neural/Processing Functions/mapminmax_reverse  xmin=0  xmax=0.989999999999999991118215802999  ymin=-1  ymax=1
      settings: SourceProductName=Deep Learning Toolbox
  y : Outport  PortDimensions=1
      mask Display: e = 0.06;c1 = [120 230 180]/255;c2 = ([120 230 180]+0)/(256+128);c3 = ([120 230 180]+128)/(256+128);patch([0 1 1 0],[0 0 1 1],c1);patch([0 1 1 1-e 1-e 0+e],[0 0 1 1-e 0+e 0+e],c2);patch([0 0 1 1-e 0+e 0+e],[0 1 1 1-e 1-e 0+e],c3);plot([0 1 1 0 0],[0 0 1 1 0]);
  wires:
  mapminmax_reverse/1 -> y/1
  a/1 -> mapminmax_reverse/1

== system ControlComparison/Control scheme/Neural MPPT Control Scheme/Mapped Duty Cycle Neural Controller/Layer 1/Delays 1 ==
  "p{1}" : Inport  PortDimensions=3
      mask Display: e = 0.06;c1 = [120 230 180]/255;c2 = ([120 230 180]+0)/(256+128);c3 = ([120 230 180]+128)/(256+128);patch([0 1 1 0],[0 0 1 1],c1);patch([0 1 1 1-e 1-e 0+e],[0 0 1 1-e 0+e 0+e],c2);patch([0 0 1 1-e 0+e 0+e],[0 1 1 1-e 1-e 0+e],c3);plot([0 1 1 0 0],[0 0 1 1 0]);
  mux : Mux  Inputs=1
      mask Display: e = 0.06;c1 = [120 150 230]/255;c2 = ([120 150 230]+0)/383;c3 = ([120 150 230]+128)/383;patch([0 1 1 0],[0 0 1 1],c1);patch([0 1 1 1-e 1-e 0+e],[0 0 1 1-e 0+e 0+e],c2);patch([0 0 1 1-e 0+e 0+e],[0 1 1 1-e 1-e 0+e],c3);plot([0 1 1 0 0],[0 0 1 1 0]);disp('Mux')
  "pd{1,1}" : Outport
      mask Display: e = 0.06;c1 = [120 230 180]/255;c2 = ([120 230 180]+0)/(256+128);c3 = ([120 230 180]+128)/(256+128);patch([0 1 1 0],[0 0 1 1],c1);patch([0 1 1 1-e 1-e 0+e],[0 0 1 1-e 0+e 0+e],c2);patch([0 0 1 1-e 0+e 0+e],[0 1 1 1-e 1-e 0+e],c3);plot([0 1 1 0 0],[0 0 1 1 0]);
  wires:
  mux/1 -> "pd{1,1}"/1
  "p{1}"/1 -> mux/1
